simulink model "PA11_7_sim"  (R2024a)
settings: Solver=ode4  StartTime=0.0  StopTime=10.0  FixedStep=0.01  RelTol=1e-3
values from neighbouring files (symbols this model uses):
  A = [-10, 1, 0; -16, 0, 1; 0, 0, 0]    [PA11_7.m]
  B = [0; 0; 120]    [PA11_7.m]
  K = acker(A, B, p)    [PA11_7.m]
settings Model: Creator=caugu  LastModifiedBy=caugu

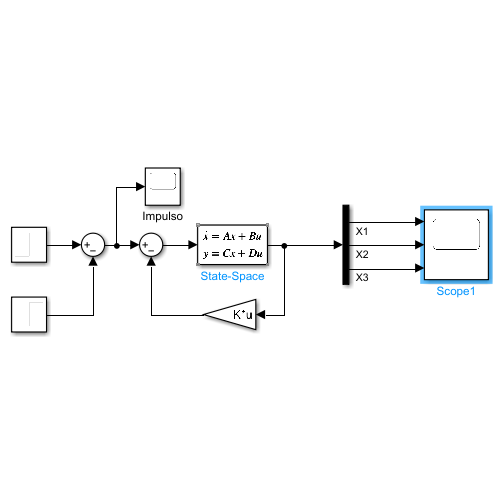
[thumbnail: Simulink's stored preview of the top-level diagram]
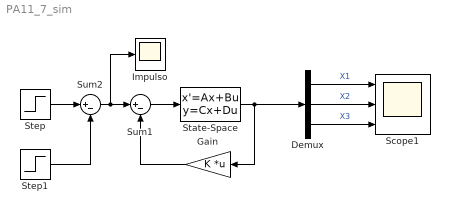
== system PA11_7_sim ==
  Demux : Demux  Outputs=3
  Gain : Gain  Gain=K  Multiplication=Matrix(K*u)
  Impulso : Scope
  Scope1 : Scope  NumInputPorts=3
  State-Space : StateSpace  A=A  B=B  C=eye(3)  D=zeros(3,1)  InitialCondition=0
  Step : Step  After=10  SampleTime=0
  Step1 : Step  Time=1.05  After=10  SampleTime=0
  Sum1 : Sum  Inputs=|+-
  Sum2 : Sum  Inputs=|+-
  wires:
  Gain/1 -> Sum1/2
  State-Space/1 -> Demux/1, Gain/1
  Sum1/1 -> State-Space/1
  Step/1 -> Sum2/1
  Step1/1 -> Sum2/2
  Demux/1 -> Scope1/1  "X1"
  Demux/3 -> Scope1/3  "X3"
  Demux/2 -> Scope1/2  "X2"
  Sum2/1 -> Sum1/1, Impulso/1
